simulink model "sim_InvJacControl"  (R2020a)
settings: Solver=VariableStepAuto  StartTime=0.0  StopTime=T(end)  RelTol=1e-3
values from neighbouring files (symbols this model uses):
  q0 = zeros(1,NLinks)    [RobotPlot.m]
undefined symbols (not defined in the file or in its folder): B_accel, Bddq, C_q, dJacobA, Fv_dq, fwdkin, G_q, Ja_inv, Jadq, Kd, Kp, NLinks, T_step
settings Model: SimulationMode=accelerator  Creator=Dallas  LastModifiedBy=Dallas
settings DataIOCC: SaveOutput=off  ReturnWorkspaceOutputs=off

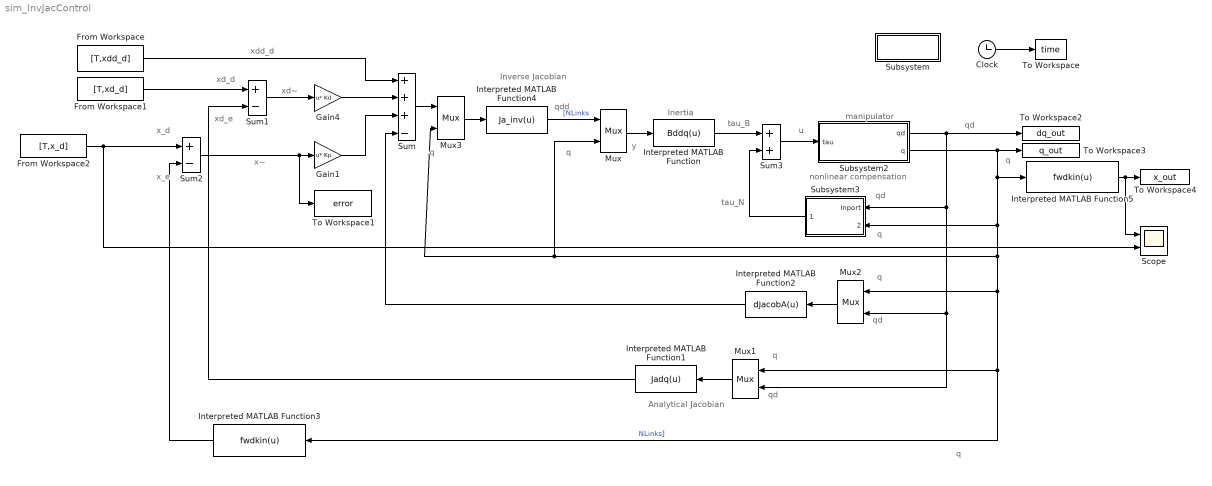
== system sim_InvJacControl ==
  note: tau_N
  note: tau_B
  note: u
  note: x_e
  note: Inertia
  note: y
  note: Analytical
      | Jacobian
  note: x~
  note: nonlinear
      | compensation
  note: Inverse
      | Jacobian
  note: manipulator
  note: xdd_d
  note: xd_e
  note: x_d
  note: xd_d
  note: xd~
  note: q
  note: q
  note: q
  note: qd
  note: qd
  note: q
  note: q
  note: qd
  note: qd
  note: q
  note: q
  note: qdd
  Clock : Clock
  From Workspace : FromWorkspace  VariableName=[T,xdd_d]  SampleTime=T_step
  From Workspace1 : FromWorkspace  VariableName=[T,xd_d]  SampleTime=T_step
  From Workspace2 : FromWorkspace  VariableName=[T,x_d]  SampleTime=T_step
  Gain1 : Gain  Gain=Kp  Multiplication=Matrix(u*K)  SampleTime=T_step
      mask Display: disp('Kp')
  Gain4 : Gain  Gain=Kd  Multiplication=Matrix(u*K)  SampleTime=T_step
      mask Display: disp('Kd')
  Interpreted MATLAB Function : MATLABFcn  MATLABFcn=Bddq(u)  OutputDimensions=NLinks
      mask Display: disp('B(q)*ddq')
  Interpreted MATLAB Function1 : MATLABFcn  MATLABFcn=Jadq(u)  OutputDimensions=3
      mask Display: disp('J(q)*dq')
  Interpreted MATLAB Function2 : MATLABFcn  MATLABFcn=dJacobA(u)  OutputDimensions=3
      mask Display: disp('dJa(q,dq)')
  Interpreted MATLAB Function3 : MATLABFcn  MATLABFcn=fwdkin(u)  OutputDimensions=3
      mask Display: disp('Fwd Kinematics (q)')
  Interpreted MATLAB Function4 : MATLABFcn  MATLABFcn=Ja_inv(u)  OutputDimensions=NLinks
      mask Display: disp('inv(Ja(q)')
  Interpreted MATLAB Function5 : MATLABFcn  MATLABFcn=fwdkin(u)  OutputDimensions=3
      mask Display: disp('Fwd Kinematics (q)')
  Mux : Mux  Inputs=[NLinks,NLinks]
  Mux1 : Mux  Inputs=[NLinks,NLinks]
  Mux2 : Mux  Inputs=[NLinks,NLinks]
  Mux3 : Mux  Inputs=[3,NLinks]
  Scope : Scope  NumInputPorts=2
  Subsystem : Subsystem  StopFcn=SimPlots
      mask Display: disp('Plot')
  Subsystem2 : Subsystem
      mask Display: disp('inv(B(q))*(tau-tau'')')
  Subsystem3 : Subsystem
      mask Display: disp('N(q,dq)')
  Sum : Sum  Inputs=+++-
  Sum1 : Sum  Inputs=+-
  Sum2 : Sum  Inputs=+-
  Sum3 : Sum
  To Workspace : ToWorkspace  VariableName=time  SampleTime=-1
      mask Display: disp('time')
  To Workspace1 : ToWorkspace  VariableName=error  SampleTime=T_step
      mask Display: disp('error')
  To Workspace2 : ToWorkspace  VariableName=dq_out  SampleTime=T_step
      mask Display: disp('dq_out')
  To Workspace3 : ToWorkspace  VariableName=q_out  SampleTime=T_step
      mask Display: disp('q_out')
  To Workspace4 : ToWorkspace  VariableName=x_out  SampleTime=T_step
      mask Display: disp('x_out')
  wires:
  From Workspace1/1 -> Sum1/1
  Sum1/1 -> Gain4/1
  Gain4/1 -> Sum/2
  From Workspace/1 -> Sum/1
  From Workspace2/1 -> Scope/2, Sum2/1
  Interpreted MATLAB Function1/1 -> Sum1/2
  Subsystem2/2(q) -> Subsystem3/2(Inport1), Mux/2, Mux3/2, Mux2/1, Mux1/1, Interpreted MATLAB Function3/1, Interpreted MATLAB Function5/1, To Workspace3/1  "NLinks]"
  Interpreted MATLAB Function/1 -> Sum3/1
  Sum3/1 -> Subsystem2/1(tau)
  Subsystem2/1(qd) -> Subsystem3/1(Inport), Mux1/2, Mux2/2, To Workspace2/1
  Subsystem3/1(Outport) -> Sum3/2
  Sum2/1 -> To Workspace1/1, Gain1/1
  Gain1/1 -> Sum/3
  Clock/1 -> To Workspace/1
  Interpreted MATLAB Function2/1 -> Sum/4
  Mux/1 -> Interpreted MATLAB Function/1
  Mux1/1 -> Interpreted MATLAB Function1/1
  Mux2/1 -> Interpreted MATLAB Function2/1
  Interpreted MATLAB Function3/1 -> Sum2/2
  Mux3/1 -> Interpreted MATLAB Function4/1
  Sum/1 -> Mux3/1
  Interpreted MATLAB Function4/1 -> Mux/1  "[NLinks"
  Interpreted MATLAB Function5/1 -> Scope/1, To Workspace4/1

== system sim_InvJacControl/Subsystem ==

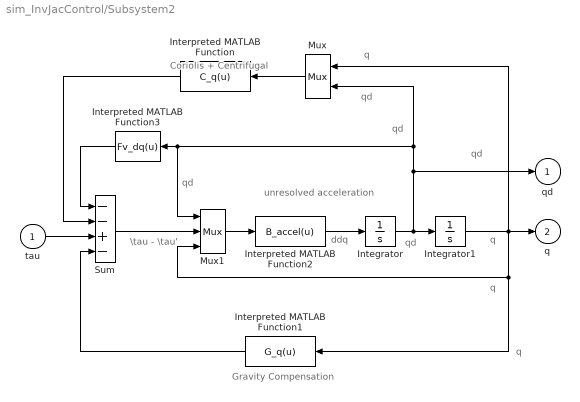
== system sim_InvJacControl/Subsystem2 ==
  note: \tau - \tau'
  note: Gravity Compensation
  note: Coriolis + Centrifugal
  note: qd
  note: q
  note: unresolved
      | acceleration
  note: q
  note: q
  note: qd
  note: qd
  note: ddq
  note: q
  note: qd
  note: qd
  tau : Inport
  Integrator : Integrator
  Integrator1 : Integrator  InitialCondition=q0
  Interpreted MATLAB Function : MATLABFcn  MATLABFcn=C_q(u)  OutputDimensions=NLinks  Output1D=off
      mask Display: disp('C(q,dq)*dq')
  Interpreted MATLAB Function1 : MATLABFcn  MATLABFcn=G_q(u)  OutputDimensions=NLinks
      mask Display: disp('G(q)')
  Interpreted MATLAB Function2 : MATLABFcn  MATLABFcn=B_accel(u)  OutputDimensions=NLinks
      mask Display: disp('ddq(q,dq,tau)')
  Interpreted MATLAB Function3 : MATLABFcn  MATLABFcn=Fv_dq(u)  OutputDimensions=NLinks
      mask Display: disp('Fv(dq)')
  Mux : Mux  Inputs=[NLinks,NLinks]
  Mux1 : Mux  Inputs=[NLinks,NLinks,NLinks]
  Sum : Sum  Inputs=--+-
  qd : Outport
  q : Outport  Port=2
  wires:
  tau/1 -> Sum/3
  Sum/1 -> Mux1/2
  Interpreted MATLAB Function2/1 -> Integrator/1
  Interpreted MATLAB Function1/1 -> Sum/4
  Integrator/1 -> Integrator1/1, Interpreted MATLAB Function3/1, Mux1/1, Mux/2, qd/1
  Interpreted MATLAB Function/1 -> Sum/2
  Interpreted MATLAB Function3/1 -> Sum/1
  Integrator1/1 -> Interpreted MATLAB Function1/1, Mux1/3, Mux/1, q/1
  Mux/1 -> Interpreted MATLAB Function/1
  Mux1/1 -> Interpreted MATLAB Function2/1

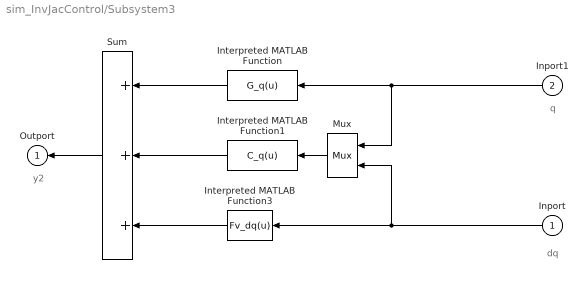
== system sim_InvJacControl/Subsystem3 ==
  note: y2
  note: dq
  note: q
  Inport : Inport
  Inport1 : Inport  Port=2
  Interpreted MATLAB Function : MATLABFcn  MATLABFcn=G_q(u)  OutputDimensions=NLinks
      mask Display: disp('G(q)')
  Interpreted MATLAB Function1 : MATLABFcn  MATLABFcn=C_q(u)  OutputDimensions=NLinks
      mask Display: disp('C(q,dq)*dq')
  Interpreted MATLAB Function3 : MATLABFcn  MATLABFcn=Fv_dq(u)  OutputDimensions=NLinks
      mask Display: disp('Fv(dq)')
  Mux : Mux  Inputs=2
  Sum : Sum  Inputs=+++
  Outport : Outport
  wires:
  Inport1/1 -> Mux/1, Interpreted MATLAB Function/1
  Inport/1 -> Interpreted MATLAB Function3/1, Mux/2
  Mux/1 -> Interpreted MATLAB Function1/1
  Interpreted MATLAB Function1/1 -> Sum/2
  Interpreted MATLAB Function3/1 -> Sum/3
  Interpreted MATLAB Function/1 -> Sum/1
  Sum/1 -> Outport/1
